simulink subsystem "subsistema_electromagnetico"  (R2023b)
settings: Solver=VariableStepAuto  StartTime=0.0  StopTime=10.0  RelTol=1e-3
settings Model: Creator=nicol  LastModifiedBy=Julya

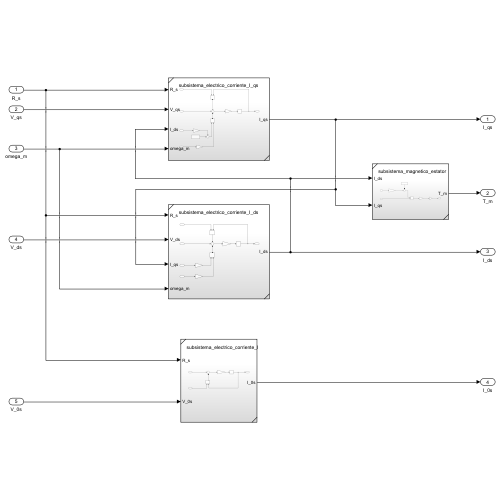
[thumbnail: Simulink's stored preview of the top-level diagram]
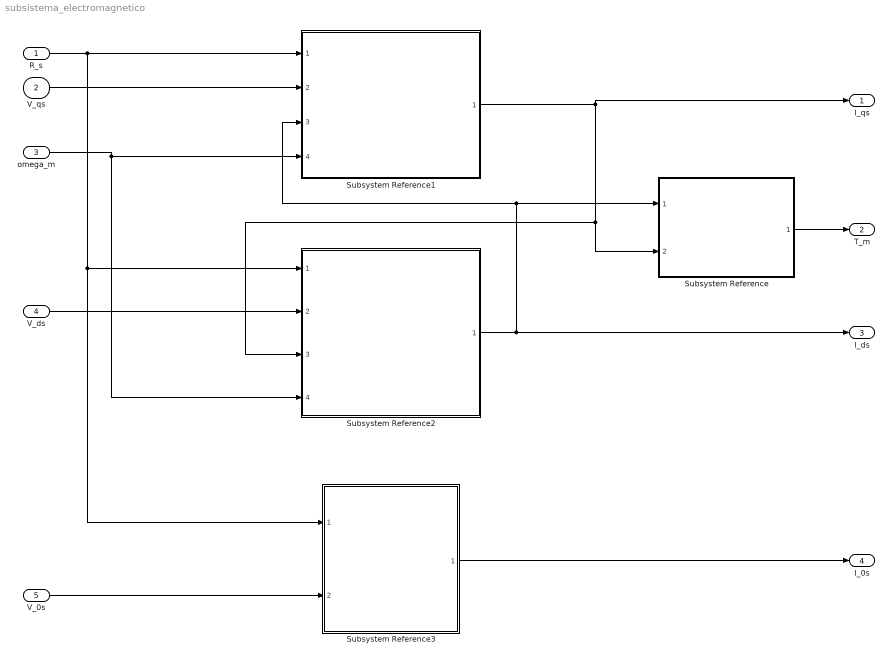
== system subsistema_electromagnetico ==
  R_s : Inport
  V_qs : Inport  Port=2
  omega_m : Inport  Port=3
  V_ds : Inport  Port=4
  V_0s : Inport  Port=5
  Subsystem Reference : Subsystem  ReferencedSubsystem=subsistema_magnetico_estator
  Subsystem Reference1 : Subsystem  ReferencedSubsystem=subsistema_electrico_corriente_I_qs
  Subsystem Reference2 : Subsystem  ReferencedSubsystem=subsistema_electrico_corriente_I_ds
  Subsystem Reference3 : Subsystem  ReferencedSubsystem=subsistema_electrico_corriente_I_0s
  I_qs : Outport
  T_m : Outport  Port=2
  I_ds : Outport  Port=3
  I_0s : Outport  Port=4
  wires:
  V_0s/1 -> Subsystem Reference3/2
  V_ds/1 -> Subsystem Reference2/2
  omega_m/1 -> Subsystem Reference2/4, Subsystem Reference1/4
  V_qs/1 -> Subsystem Reference1/2
  R_s/1 -> Subsystem Reference3/1, Subsystem Reference2/1, Subsystem Reference1/1
  Subsystem Reference2/1 -> I_ds/1, Subsystem Reference/1, Subsystem Reference1/3
  Subsystem Reference3/1 -> I_0s/1
  Subsystem Reference1/1 -> Subsystem Reference2/3, Subsystem Reference/2, I_qs/1
  Subsystem Reference/1 -> T_m/1
